simulink model "standalonefuelcell"  (R2024b)
settings: Solver=ode23tb  StartTime=0.0  StopTime=0.06  RelTol=1e-3  EnableMultiTasking=on
libraries: spsSeriesRLCBranchLib x2, spsVoltageMeasurementLib x2, spsThreePhaseVIMeasurementLib x1, spsThreePhaseSeriesRLCLoadLib x1, spsDiodeLib x1, spsMosfetLib x1, spsFuelCellStackLib x1, spsUniversalBridgeLib x1, spsMeanLib x1, spsRMSLib x1, powerlib_extras x1, spspowerguiLib x1
settings Model: Creator=GOVIND  LastModifiedBy=realm
settings SolverCC: AlgebraicLoopSolver=TrustRegion
settings DataIOCC: LimitDataPoints=on  SaveFormat=Array  SignalLoggingSaveFormat=ModelDataLogs  ReturnWorkspaceOutputs=off
settings OptimizationCC: ExpressionDepthLimit=2147483647  LifeSpan=inf
settings DebuggingCC: UnderspecifiedInitializationDetection=Classic  MergeDetectMultiDrivingBlocksExec=none  SolverPrmCheckMsg=warning  FcnCallInpInsideContextMsg=warning  UnconnectedInputMsg=warning  UnconnectedOutputMsg=warning  UnconnectedLineMsg=warning  StateNameClashWarn=warning  SFUnexpectedBacktrackingDiag=warning  SFNoUnconditionalDefaultTransitionDiag=warning  SFExecutionAtInitializationDiag=none  ArithmeticOperatorsInVariantConditions=warning
settings HardwareCC: ProdBitPerPointer=32  ProdBitPerSizeT=32  ProdBitPerPtrDiffT=32  ProdLargestAtomicFloat=None  ProdIntDivRoundTo=Undefined  ProdEndianess=Unspecified  ProdWordSize=32  ProdHWDeviceType=32-bit Generic
settings ModelReferenceCC: EnableRefExpFcnMdlSchedulingChecks=on  PropagateSignalLabelsOutOfModel=off
settings SFSimCC: SimUseLocalCustomCode=off  CustomCodeUndefinedFunction=UseInterfaceOnly
settings RTWCC: RTWUseLocalCustomCode=off  GPUComputeCapability=3.5
settings CodeAppCC: StateflowObjectComments=on
settings GRTTargetCC: TargetLangStandard=C89/C90 (ANSI)  CombineOutputUpdateFcns=off  GRTInterface=on
settings ConfigComp: CovMetricSettings=dw  CovSaveCumulativeToWorkspaceVar=on  CovSaveSingleToWorkspaceVar=on  CovExternalEMLEnable=off

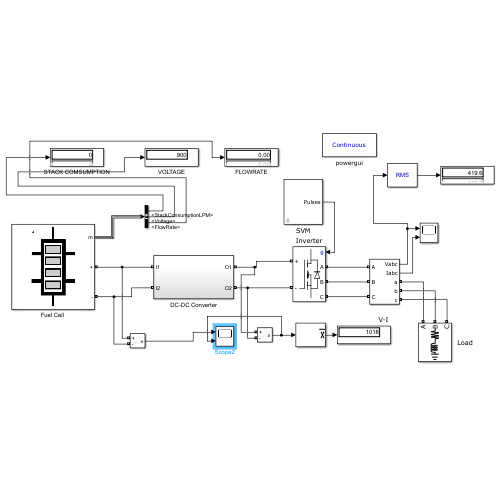
[thumbnail: Simulink's stored preview of the top-level diagram]
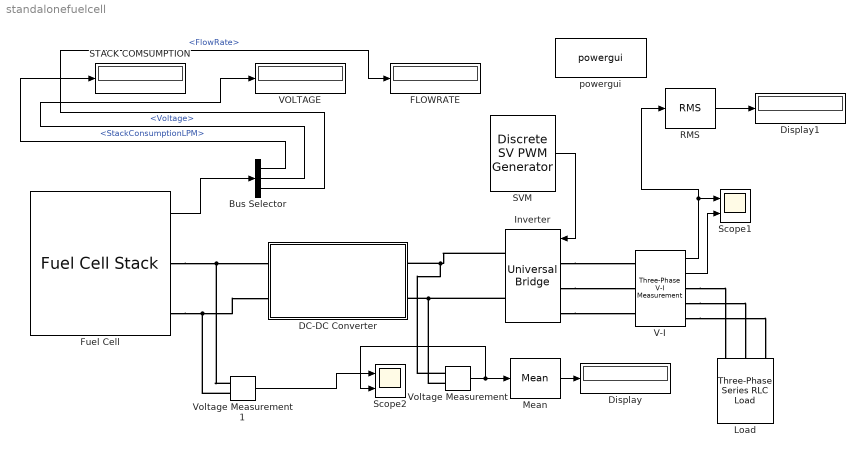
== system standalonefuelcell ==
  " V-I " : spsThreePhaseVIMeasurementLib/Three-Phase V-I Measurement  VoltageMeasurement=phase-to-ground  SetLabelV=off  LabelV=Vabc  Vpu=off  VpuLL=off  CurrentMeasurement=yes  SetLabelI=off  LabelI=Iabc  Ipu=off  Pbase=100e6  Vbase=500e3  OutputType=Complex  PhasorSimulation=off  PSBequivalent=0
  " Load" : spsThreePhaseSeriesRLCLoadLib/Three-Phase Series RLC Load  LConnTagsString=A|B|C  Configuration=Y (grounded)  NominalVoltage=500  Vabc=[1e3 1e3 1e3]  Vabcp=[1e3 1e3 1e3]  NominalFrequency=50  UnbalancedPower=off  ActivePower=500  InductivePower=100  CapacitivePower=0  Pabc=[10e3 9e3 11e3]  QLabc=[100 90 110]  QCabc=[100 90 110]  Pabcp=[10e3 9e3 11e3]  QLabcp=[100 90 110]  QCabcp=[100 90 110]  Measurements=None  LoadType=constant Z
  Bus Selector : BusSelector  OutputSignals=StackConsumptionLPM,Voltage,FlowRate
  DC-DC Converter : Subsystem
  Display : Display
  Display1 : Display
  FLOWRATE : Display
      settings: Format=bank
  "Fuel Cell " : spsFuelCellStackLib/Fuel Cell Stack  PresetModel=PEMFC - 50 kW - 625 Vdc  FcType=Proton Exchange Membrane (PEM)  Detailed=Simplified  Eoc=[900,895]  NomVI=[80,625]  EndVI=[280,430]  Nc=900  n=55  TOp=65  AirFr=2100  SuppPress=[1.5,1]  Comp=[99.95,21,1]  SignX=off  SignY=off  FlowRateH2=on  FlowRateAir=off  SystemTemp=off  SystemPH2=off  SystemPAir=off  FCDyn=off  FC_tau=0  Peak_O2=80  V_Under=10
  Inverter : spsUniversalBridgeLib/Universal Bridge  Arms=3  SnubberResistance=1e5  SnubberCapacitance=inf  Device=MOSFET / Diodes  Ron=1e-3  Lon=0  ForwardVoltages="[  0  0  ]"  ForwardVoltage=0  GTOparameters=[ 10e-6 , 20e-6 ]  IGBTparameters=[ 1e-6 , 2e-6 ]  Measurements=None  Measurements_2=None  converterType=Rectifier
  Mean : spsMeanLib/Mean  Freq=60  Vinit=0  Ts=0
  RMS : spsRMSLib/RMS  TrueRMS=on  Freq=50  RMSInit=120  Ts=0
  STACK COMSUMPTION : Display
      settings: Decimation=5
  SVM : powerlib_extras/Discrete  Control Blocks/Discrete SV PWM Generator  InputType=Internally generated  SwitchingPattern=Pattern #1  Fc=10000  ParUref=[0.8 0 50]  Ts=2e-6
  Scope1 : Scope  NumInputPorts=2
  Scope2 : Scope  NumInputPorts=2
  VOLTAGE : Display
  Voltage Measurement : spsVoltageMeasurementLib/Voltage Measurement  PhasorSimulation=off  OutputType=Complex  PSBequivalent=0
  Voltage Measurement1 : spsVoltageMeasurementLib/Voltage Measurement  PhasorSimulation=off  OutputType=Complex  PSBequivalent=0
  powergui : spspowerguiLib/powergui  Priority=1  SimulationMode=Continuous  SampleTime=50e-6  frequency=50  Iterations=50  frequencyindice=0  Pbase=100e6  ErrMax=1e-4  UnitsV=kV  UnitsW=MW  buscounter=0  FunctionMessages=off  echomessages=off  EnableUseOfTLC=off  CurrentSourceSwitches=off  DisableSnubberDevices=off  DisableRonSwitches=off  DisableVfSwitches=off  DisplayEquations=off  AutomaticDiscreteSolvers=off  SolverType=Tustin/Backward Euler (TBE)  Interpol=off  ExternalGateDelay=off  methode=off  Ts=0  x0status=blocks  SPID=off  SwTol=0  HookPort=off  NonlinearTolerance=1e-4  nMaxIteration=100  ContinueOnMaxIteration=off  RestoreLinks=warning  ResistiveCurrentMeasurement=off  Frange=[0:2:500]  Ylog=off  Xlog=on  ShowGrid=off  save=off  variable=ZData  structure=simout2  ZoomFFT=on  StartTime=0.02  cycles=2  DisplayStyle=1  fundamental=50  FreqAxis=on  MaxFrequency=5000  frequencyindicesteady=1  RmsSteady=1  display=off
  wires:
  " V-I "/1 -> RMS/1, Scope1/1
  " V-I "/2 -> Scope1/2
  SVM/1 -> Inverter/1
  "Fuel Cell "/1 -> Bus Selector/1
  Bus Selector/1 -> STACK COMSUMPTION/1  "<StackConsumptionLPM>"
  Bus Selector/2 -> VOLTAGE/1  "<Voltage>"
  Bus Selector/3 -> FLOWRATE/1  "<FlowRate>"
  Voltage Measurement/1 -> Scope2/2, Mean/1
  Mean/1 -> Display/1
  Voltage Measurement1/1 -> Scope2/1
  RMS/1 -> Display1/1
  connections:
  " V-I "/RConn1 -- " Load"/LConn1
  " V-I "/RConn2 -- " Load"/LConn2
  " V-I "/RConn3 -- " Load"/LConn3
  Inverter/LConn1 -- " V-I "/LConn1
  Inverter/LConn2 -- " V-I "/LConn2
  Inverter/LConn3 -- " V-I "/LConn3
  "Fuel Cell "/RConn1 -- Voltage Measurement1/LConn1 -- DC-DC Converter/RConn1
  Inverter/RConn1 -- Voltage Measurement/LConn1 -- DC-DC Converter/LConn1
  Inverter/RConn2 -- Voltage Measurement/LConn2 -- DC-DC Converter/LConn2
  "Fuel Cell "/RConn2 -- Voltage Measurement1/LConn2 -- DC-DC Converter/RConn2

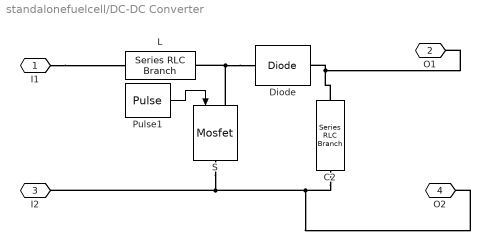
== system standalonefuelcell/DC-DC Converter ==
  C2 : spsSeriesRLCBranchLib/Series RLC Branch  LConnTagsString=__new0  RConnTagsString=__new0  BranchType=C  Resistance=1  Inductance=1e-3  SetiL0=off  InitialCurrent=0  Capacitance=2200e-6  Setx0=off  InitialVoltage=0  Measurements=None
  Diode : spsDiodeLib/Diode  Ron=0.001  Lon=0  Vf=0.8  IC=0  UseSnubber=off  Rs=500  Cs=250e-9  Measurements=off
  L : spsSeriesRLCBranchLib/Series RLC Branch  LConnTagsString=__new0  RConnTagsString=__new0  BranchType=L  Resistance=1  Inductance=10e-3  SetiL0=off  InitialCurrent=0  Capacitance=1e-6  Setx0=off  InitialVoltage=0  Measurements=None
  Pulse1 : DiscretePulseGenerator  PulseType=Time based  Amplitude=12  Period=10e-6  PulseWidth=6e-6
  S : spsMosfetLib/Mosfet  Ron=0.1  Lon=0  Rd=0.01  Vfd=0  IC=0  Rs=1e5  Cs=inf  Measurements=off
  I1 : PMIOPort  Side=Right
  O1 : PMIOPort  Port=2  Side=Left
  I2 : PMIOPort  Port=3  Side=Right
  O2 : PMIOPort  Port=4  Side=Left
  wires:
  Pulse1/1 -> S/1
  connections:
  I1/RConn1 -- L/LConn1
  O2/RConn1 -- C2/RConn1 -- I2/RConn1 -- S/RConn1
  O1/RConn1 -- C2/LConn1 -- Diode/RConn1
  Diode/LConn1 -- L/RConn1 -- S/LConn1
